simulink model "acceleration_model"  (R2024b)
settings: Solver=VariableStepAuto  StartTime=0.0  StopTime=20  RelTol=1e-3
undefined symbols (not defined in the file or in its folder): A, c_w, eta, F_R, i_A, i_G4, i_G5, m, r_R, rho, v_0
settings Model: Creator=kavin  LastModifiedBy=kavin

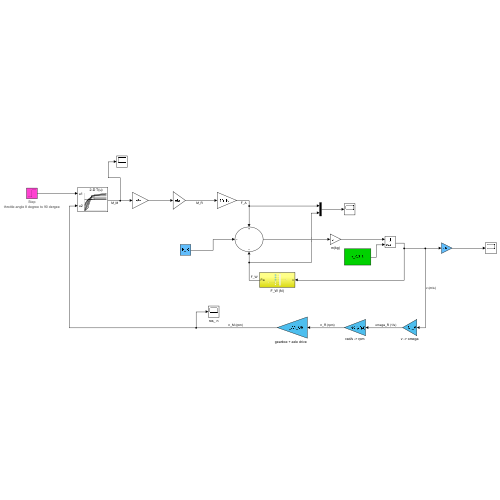
[thumbnail: Simulink's stored preview of the top-level diagram]
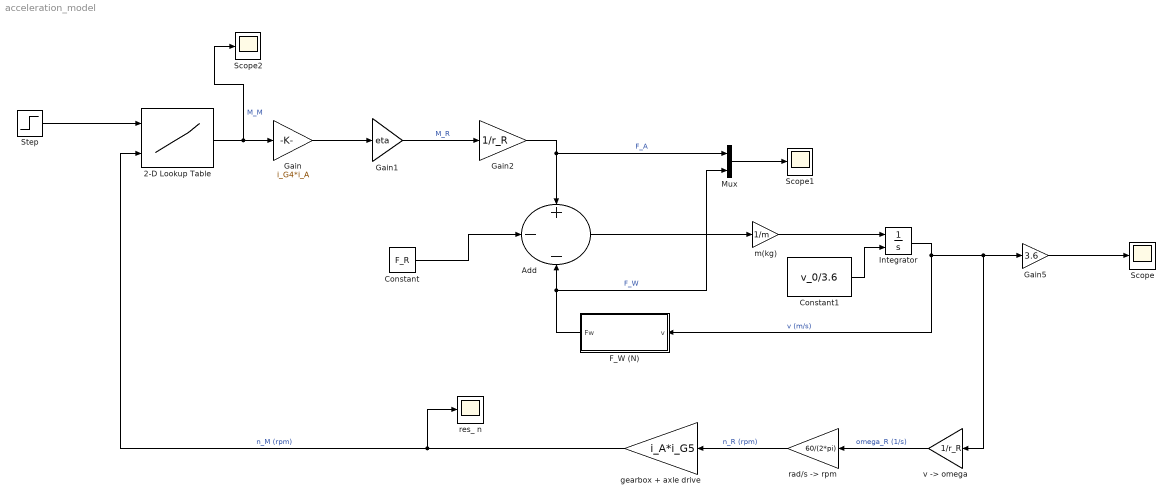
== system acceleration_model ==
  2-D Lookup Table : Lookup_n-D  BreakpointsForDimension1=cm_engine(2:end,1)  BreakpointsForDimension2=cm_engine(1,2:end)  Table=cm_engine(2:end,2:end)  InternalRulePriority=Speed  RndMeth=Simplest
      settings: InputPortMap=u0,u1
  Add : Sum  Inputs=+--
  Constant : Constant  Value=F_R
  Constant1 : Constant  Value=v_0/3.6
  F_W (N) : Subsystem
  Gain : Gain  Gain=i_G4*i_A
  Gain1 : Gain  Gain=eta
  Gain2 : Gain  Gain=1/r_R
  Gain5 : Gain  Gain=3.6
  Integrator : Integrator  InitialConditionSource=external
  Mux : Mux  Inputs=2
  Scope : Scope
  Scope1 : Scope
  Scope2 : Scope
  Step : Step  Time=5  Before=8  After=90  SampleTime=0
      settings: AttributesFormatString=|
      | %<BlockType>
      | throttle angle 8 degree to 90 dergee
  "gearbox + axle drive   " : Gain  Gain=i_A*i_G5
  m(kg) : Gain  Gain=1/m
  "rad/s -> rpm" : Gain  Gain=60/(2*pi)
  res_ n : Scope
  "v -> omega" : Gain  Gain=1/r_R
  wires:
  Step/1 -> 2-D Lookup Table/1
  2-D Lookup Table/1 -> Scope2/1, Gain/1  "M_M"
  Gain/1 -> Gain1/1
  Gain1/1 -> Gain2/1  "M_R"
  Gain2/1 -> Add/1, Mux/1  "F_A"
  F_W (N)/1(Fw) -> Mux/2, Add/3  "F_W"
  Constant/1 -> Add/2
  Add/1 -> m(kg)/1
  m(kg)/1 -> Integrator/1
  Constant1/1 -> Integrator/2
  Gain5/1 -> Scope/1
  "rad/s -> rpm"/1 -> "gearbox + axle drive   "/1  "n_R (rpm)"
  "v -> omega"/1 -> "rad/s -> rpm"/1  "omega_R (1/s)"
  Integrator/1 -> "v -> omega"/1, Gain5/1, F_W (N)/1(v)  "v (m/s)"
  "gearbox + axle drive   "/1 -> 2-D Lookup Table/2, res_ n/1  "n_M (rpm)"
  Mux/1 -> Scope1/1

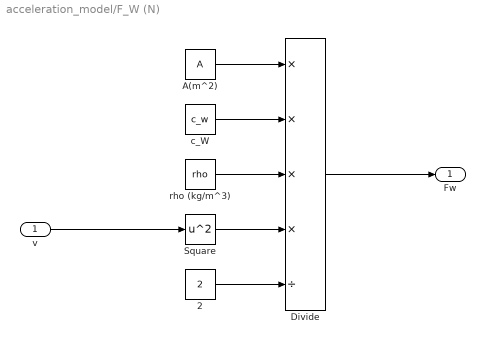
== system acceleration_model/F_W (N) ==
  v : Inport
  2 : Constant  Value=2
  A(m^2) : Constant  Value=A
  Divide : Product  Inputs=****/
  Square : Math  Operator=square
  c_W : Constant  Value=c_w
  rho (kg/m^3) : Constant  Value=rho
  Fw : Outport
  wires:
  c_W/1 -> Divide/2
  A(m^2)/1 -> Divide/1
  2/1 -> Divide/5
  Divide/1 -> Fw/1
  rho (kg/m^3)/1 -> Divide/3
  v/1 -> Square/1
  Square/1 -> Divide/4
